simulink model "findAxis"  (R2021a)
settings: Solver=FixedStepDiscrete  StartTime=0.0  StopTime=T_end*3  FixedStep=T_sim  RelTol=1e-3
values from neighbouring files (symbols this model uses):
  B = 0.00000001    (= 1e-08)    [speedControlInit.m]
  I_dref = 0    [speedControlInit.m]
  J = 0.008    [speedControlInit.m]
  mask_Ld = 52.9e-6    (= 5.29e-05)    [speedControlInit.m]
  mask_Lq = 52.9e-6    (= 5.29e-05)    [speedControlInit.m]
  mask_p = 8    [speedControlInit.m]
  mask_R_s = 45e-3    (= 0.045)    [speedControlInit.m]
  mask_Tsw = 1/F_sw    (= 2e-05)    [speedControlInit.m]
  mask_VDC = 250    [speedControlInit.m]
  PWM_INVERTER = 1    [speedControlInit.m]
  T_end = 0.5    [speedControlInit.m]
  T_sim = 1/(F_sw*100)    (= 2e-07)    [speedControlInit.m]
libraries: spsIdealSwitchLib x8, spsCurrentMeasurementLib x3, simulink x3, spsVoltageMeasurementLib x3, spsDCVoltageSourceLib x1, spsPermanentMagnetSynchronousMachineLib x1, spspowerguiLib x1
settings Model: Creator=Nishanth  LastModifiedBy=Nishanth

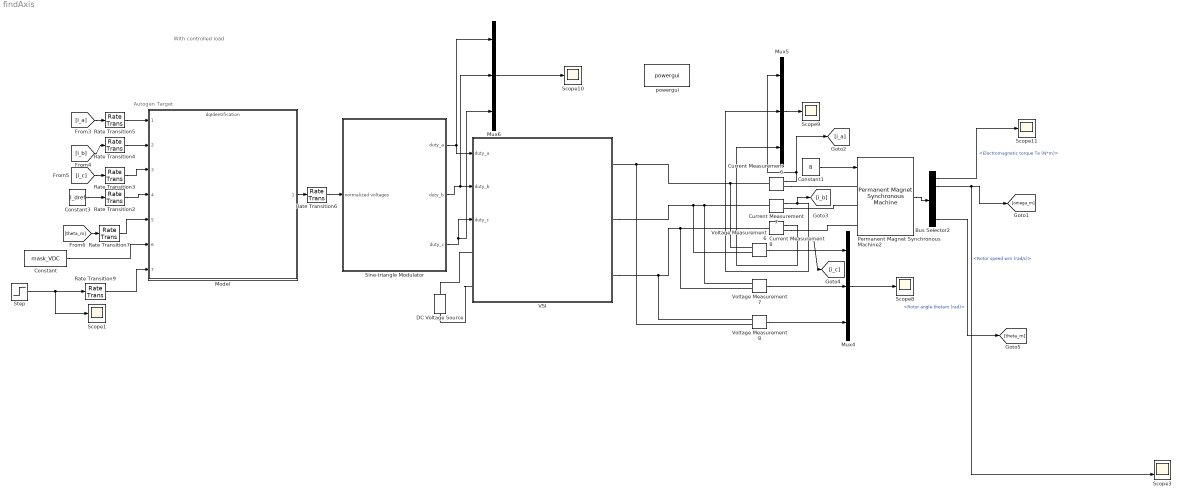
== system findAxis ==
  note: With controlled load
  note: Autogen Target
  Bus Selector2 : BusSelector  OutputSignals=Electromagnetic torque Te (N*m),Rotor speed wm (rad/s),Stator current is_a (A),Stator current is_b (A),Stator current is_c (A),Rotor angle thetam (rad)
  Constant : Constant  Value=mask_VDC
  Constant1 : Constant  Value=8
  Constant3 : Constant  Value=I_dref
  Current Measurement6 : spsCurrentMeasurementLib/Current Measurement  PhasorSimulation=off  OutputType=Complex  PSBequivalent=0
  Current Measurement7 : spsCurrentMeasurementLib/Current Measurement  PhasorSimulation=off  OutputType=Complex  PSBequivalent=0
  Current Measurement8 : spsCurrentMeasurementLib/Current Measurement  PhasorSimulation=off  OutputType=Complex  PSBequivalent=0
  DC Voltage Source : spsDCVoltageSourceLib/DC Voltage Source  Amplitude=mask_VDC  Measurements=None
  Model : ModelReference  ModelNameDialog=dqIdentification.slx  SimulationMode=Normal  ModelReferenceVersion=2.39
  Mux4 : Mux  Inputs=3
  Mux5 : Mux  Inputs=3
  Mux6 : Mux  Inputs=3
  Permanent Magnet Synchronous Machine2 : spsPermanentMagnetSynchronousMachineLib/Permanent Magnet Synchronous Machine  NbPhases=3  FluxDistribution=Sinusoidal  RotorType=Salient-pole  MechanicalLoad=Torque Tm  PresetModel=No  ShowDetailedParameters=on  MeasurementBus=off  Resistance=mask_R_s  Inductance=8.5e-3  dqInductances=[mask_Ld, mask_Lq]  La=0.000061  MachineConstant=Torque Constant (N.m / A_peak)  Flux=0.0105  VoltageCst=15.2359  TorqueCst=mask_Kt  Flat=120  Mechanical=[J B mask_p 0]  PolePairs=mask_p  InitialConditions=[0,0, 0,0]  InitialConditions5ph=[0 0 0 0 0 0]  RefAngle=Aligned with phase A axis (original Park)  IterativeDiscreteModel=Trapezoidal non iterative  TsBlock=-1  TsPowergui=0
  Rate Transition{2..7,9} (7 alike) : RateTransition  OutPortSampleTime=mask_Ts
  Scope{1,8..11} (5 alike) : Scope
  Scope3 : Scope  NumInputPorts=2
  Sine-triangle Modulator : Subsystem
  Step : Step  Time=T_end/4  After=10  SampleTime=0
  VSI : Subsystem
  Voltage Measurement6 : spsVoltageMeasurementLib/Voltage Measurement  PhasorSimulation=off  OutputType=Complex  PSBequivalent=0
  Voltage Measurement7 : spsVoltageMeasurementLib/Voltage Measurement  PhasorSimulation=off  OutputType=Complex  PSBequivalent=0
  Voltage Measurement8 : spsVoltageMeasurementLib/Voltage Measurement  PhasorSimulation=off  OutputType=Complex  PSBequivalent=0
  powergui : spspowerguiLib/powergui  Priority=1  SimulationMode=Discrete  SampleTime=T_sim  frequency=60  Iterations=50  frequencyindice=0  Pbase=100e6  ErrMax=1e-4  UnitsV=kV  UnitsW=MW  buscounter=0  FunctionMessages=off  echomessages=off  EnableUseOfTLC=off  CurrentSourceSwitches=off  DisableSnubberDevices=off  DisableRonSwitches=off  DisableVfSwitches=off  DisplayEquations=off  AutomaticDiscreteSolvers=off  SolverType=Tustin/Backward Euler (TBE)  Interpol=off  ExternalGateDelay=off  methode=off  Ts=100  x0status=blocks  SPID=on  SwTol=0  HookPort=off  NonlinearTolerance=1e-4  nMaxIteration=100  ContinueOnMaxIteration=off  RestoreLinks=warning  ResistiveCurrentMeasurement=off  Frange=[0:2:500]  Ylog=off  Xlog=on  ShowGrid=off  save=off  variable=ZData  structure=0  ZoomFFT=off  StartTime=0.0  cycles=1  DisplayStyle=1  fundamental=60  FreqAxis=off  MaxFrequency=1000  frequencyindicesteady=1  RmsSteady=1  display=off
  wires:
  Bus Selector2/2 -> Scope3/2, [omega_m]  "<Rotor speed wm (rad/s)>"
  Voltage Measurement7/1 -> Mux4/2
  Voltage Measurement6/1 -> Mux4/1
  Bus Selector2/1 -> Scope11/1  "<Electromagnetic torque Te (N*m)>"
  Permanent Magnet Synchronous Machine2/1 -> Bus Selector2/1
  Current Measurement7/1 -> [i_b], Mux5/2
  Current Measurement8/1 -> [i_c], Mux5/3
  Voltage Measurement8/1 -> Mux4/3
  Current Measurement6/1 -> Mux5/1, [i_a]
  Mux4/1 -> Scope8/1
  Mux5/1 -> Scope9/1
  Constant1/1 -> Permanent Magnet Synchronous Machine2/1
  Rate Transition3/1 -> Model/3
  Rate Transition6/1 -> Sine-triangle Modulator/1(normalized voltages)
  Model/1 -> Rate Transition6/1
  [i_c] -> Rate Transition3/1
  [i_b] -> Rate Transition4/1
  [i_a] -> Rate Transition5/1
  Rate Transition5/1 -> Model/1
  Sine-triangle Modulator/1(duty_a) -> VSI/1(duty_a), Mux6/1
  Rate Transition2/1 -> Model/4
  Rate Transition4/1 -> Model/2
  Constant3/1 -> Rate Transition2/1
  [theta_m] -> Rate Transition7/1
  Mux6/1 -> Scope10/1
  Sine-triangle Modulator/2(duty_b) -> Mux6/2, VSI/2(duty_b)
  Sine-triangle Modulator/3(duty_c) -> Mux6/3, VSI/3(duty_c)
  Bus Selector2/6 -> [theta_m]  "<Rotor angle thetam (rad)>"
  Step/1 -> Scope1/1, Rate Transition9/1
  Rate Transition7/1 -> Model/5
  Constant/1 -> Model/6
  Rate Transition9/1 -> Model/7
  connections:
  DC Voltage Source/RConn1 -- VSI/LConn1
  VSI/LConn2 -- DC Voltage Source/LConn1
  Current Measurement6/LConn1 -- Voltage Measurement6/LConn1 -- Voltage Measurement8/LConn2 -- VSI/RConn1
  VSI/RConn2 -- Voltage Measurement6/LConn2 -- Voltage Measurement7/LConn1 -- Current Measurement7/LConn1
  VSI/RConn3 -- Voltage Measurement8/LConn1 -- Voltage Measurement7/LConn2 -- Current Measurement8/LConn1
  Current Measurement8/RConn1 -- Permanent Magnet Synchronous Machine2/LConn3
  Current Measurement7/RConn1 -- Permanent Magnet Synchronous Machine2/LConn2
  Current Measurement6/RConn1 -- Permanent Magnet Synchronous Machine2/LConn1

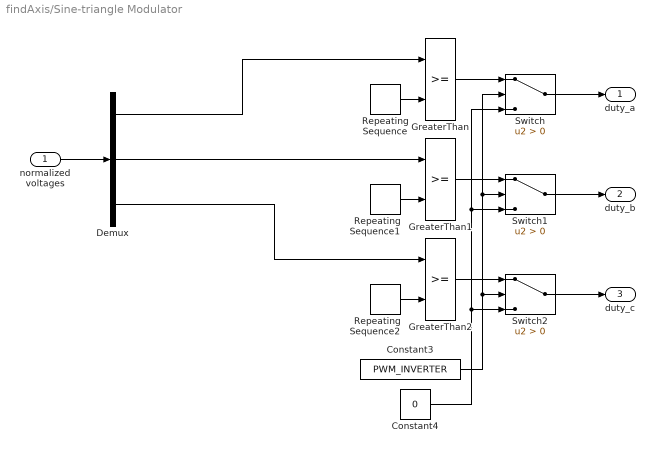
== system findAxis/Sine-triangle Modulator ==
  normalized voltages : Inport
  Constant3 : Constant  Value=PWM_INVERTER
  Constant4 : Constant  Value=0
  Demux : Demux  Outputs=3
  GreaterThan : RelationalOperator  OutDataTypeStr=boolean  RndMeth=Simplest
  GreaterThan1 : RelationalOperator  OutDataTypeStr=boolean  RndMeth=Simplest
  GreaterThan2 : RelationalOperator  OutDataTypeStr=boolean  RndMeth=Simplest
  Repeating Sequence : simulink/Sources/Repeating Sequence  rep_seq_t=[0 mask_Tsw/2 mask_Tsw]  rep_seq_y=[-1 1 -1]
  Repeating Sequence1 : simulink/Sources/Repeating Sequence  rep_seq_t=[0 mask_Tsw/2 mask_Tsw]  rep_seq_y=[-1 1 -1]
  Repeating Sequence2 : simulink/Sources/Repeating Sequence  rep_seq_t=[0 mask_Tsw/2 mask_Tsw]  rep_seq_y=[-1 1 -1]
  Switch : Switch  Criteria=u2 > Threshold
  Switch1 : Switch  Criteria=u2 > Threshold
  Switch2 : Switch  Criteria=u2 > Threshold
  duty_a : Outport
  duty_b : Outport  Port=2
  duty_c : Outport  Port=3
  wires:
  GreaterThan2/1 -> Switch2/1
  GreaterThan1/1 -> Switch1/1
  GreaterThan/1 -> Switch/1
  Repeating Sequence1/1 -> GreaterThan1/2
  Constant3/1 -> Switch2/2, Switch1/2, Switch/2
  Repeating Sequence/1 -> GreaterThan/2
  Switch2/1 -> duty_c/1
  Constant4/1 -> Switch/3, Switch1/3, Switch2/3
  Switch1/1 -> duty_b/1
  Switch/1 -> duty_a/1
  Repeating Sequence2/1 -> GreaterThan2/2
  normalized voltages/1 -> Demux/1
  Demux/1 -> GreaterThan/1
  Demux/2 -> GreaterThan1/1
  Demux/3 -> GreaterThan2/1

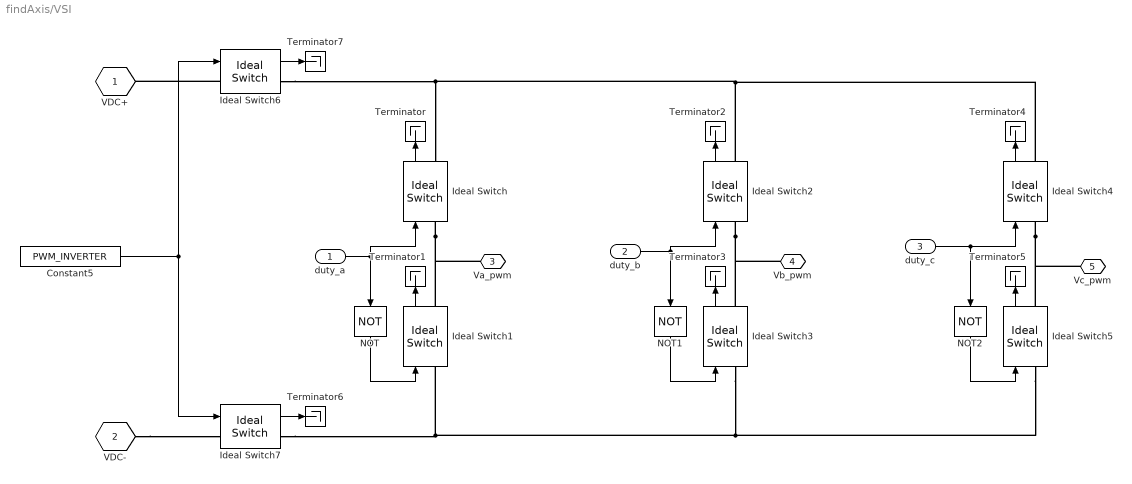
== system findAxis/VSI ==
  duty_a : Inport
  duty_b : Inport  Port=2
  duty_c : Inport  Port=3
  Constant5 : Constant  Value=PWM_INVERTER
  Ideal Switch{,1..6} (7 alike) : spsIdealSwitchLib/Ideal Switch  Ron=0.00001  Lon=0  IC=0  Rs=1e5  Cs=inf  Measurements=on
  Ideal Switch7 : spsIdealSwitchLib/Ideal Switch  Ron=0.001  Lon=0  IC=0  Rs=1e5  Cs=inf  Measurements=on
  NOT : Logic  Operator=NOT  IconShape=distinctive  AllPortsSameDT=off  OutDataTypeStr=boolean
  NOT1 : Logic  Operator=NOT  IconShape=distinctive  AllPortsSameDT=off  OutDataTypeStr=boolean
  NOT2 : Logic  Operator=NOT  IconShape=distinctive  AllPortsSameDT=off  OutDataTypeStr=boolean
  Terminator{,1..7} (8 alike) : Terminator
  VDC+ : PMIOPort  Tag=PMCPort  Side=Left
  VDC- : PMIOPort  Tag=PMCPort  Port=2  Side=Left
  Va_pwm : PMIOPort  Tag=PMCPort  Port=3  Side=Right
  Vb_pwm : PMIOPort  Tag=PMCPort  Port=4  Side=Right
  Vc_pwm : PMIOPort  Tag=PMCPort  Port=5  Side=Right
  wires:
  duty_b/1 -> Ideal Switch2/1, NOT1/1
  Ideal Switch4/1 -> Terminator4/1
  Ideal Switch/1 -> Terminator/1
  Ideal Switch2/1 -> Terminator2/1
  Ideal Switch1/1 -> Terminator1/1
  NOT/1 -> Ideal Switch1/1
  Ideal Switch5/1 -> Terminator5/1
  Ideal Switch3/1 -> Terminator3/1
  NOT2/1 -> Ideal Switch5/1
  duty_c/1 -> NOT2/1, Ideal Switch4/1
  Ideal Switch6/1 -> Terminator7/1
  duty_a/1 -> Ideal Switch/1, NOT/1
  Constant5/1 -> Ideal Switch6/1, Ideal Switch7/1
  NOT1/1 -> Ideal Switch3/1
  Ideal Switch7/1 -> Terminator6/1
  connections:
  VDC-/RConn1 -- Ideal Switch7/LConn1
  Ideal Switch2/RConn1 -- Ideal Switch6/RConn1 -- Ideal Switch/RConn1 -- Ideal Switch4/RConn1
  Ideal Switch/LConn1 -- Ideal Switch1/RConn1 -- Va_pwm/RConn1
  Ideal Switch4/LConn1 -- Ideal Switch5/RConn1 -- Vc_pwm/RConn1
  Ideal Switch2/LConn1 -- Ideal Switch3/RConn1 -- Vb_pwm/RConn1
  Ideal Switch3/LConn1 -- Ideal Switch7/RConn1 -- Ideal Switch1/LConn1 -- Ideal Switch5/LConn1
  Ideal Switch6/LConn1 -- VDC+/RConn1
